simulink model "Momentum_wheel_IP_two"  (R2024b)
settings: Solver=ode15s  StartTime=0.0  StopTime=1  RelTol=1e-3
undefined symbols (not defined in the file): X, Y, Z
libraries: sm_lib x37, nesl_utility x15, slpidlib x4
(part 2 of 2)

== matlab function Momentum_wheel_IP_two/MATLAB Function ==
  data: u input; y output; data input
function y = fcn(u, data)
if (u<5) && (u>-5)
    y=data;
else
    y=0;
end
